simulink library "dynamicsLibrary"  (R2019a)
settings: Solver=ode45  StartTime=0.0  StopTime=10.0  RelTol=1e-3  EnableMultiTasking=on
undefined symbols (not defined in the file): Vehicle
settings Model: Creator=The MathWorks, Inc.  LastModifiedBy=yahyaaba
settings DataIOCC: LimitDataPoints=on  SaveFormat=Array  ReturnWorkspaceOutputs=off
settings OptimizationCC: LifeSpan=inf
settings DebuggingCC: UnderspecifiedInitializationDetection=Classic  MergeDetectMultiDrivingBlocksExec=none  SolverPrmCheckMsg=warning  AllowSymbolicDim=off  SFUnexpectedBacktrackingDiag=warning  SFNoUnconditionalDefaultTransitionDiag=warning  SFExecutionAtInitializationDiag=none  ArithmeticOperatorsInVariantConditions=warning
settings HardwareCC: ProdBitPerPointer=32  ProdBitPerSizeT=32  ProdBitPerPtrDiffT=32  ProdLargestAtomicFloat=None  ProdIntDivRoundTo=Undefined  ProdEndianess=Unspecified  ProdWordSize=32  ProdHWDeviceType=32-bit Generic
settings ModelReferenceCC: PropagateSignalLabelsOutOfModel=off
settings SFSimCC: SimUseLocalCustomCode=off
settings RTWCC: RTWUseLocalCustomCode=off
settings CodeAppCC: StateflowObjectComments=on
settings GRTTargetCC: TargetLangStandard=C89/C90 (ANSI)  GeneratePreprocessorConditionals=Disable all
settings ConfigComp: CovMetricSettings=dw  CovHtmlReporting=on  CovSaveCumulativeToWorkspaceVar=on  CovSaveSingleToWorkspaceVar=on  CovExternalEMLEnable=off  CovSFcnEnable=off

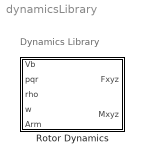
== system dynamicsLibrary ==
  note: Dynamics Library
  Rotor Dynamics : Subsystem  TreatAsAtomicUnit=on
      mask init:
      | aeroicon('aeroblk');
      settings: RTWFcnNameOpts=Use subsystem name  RTWFileNameOpts=Use function name

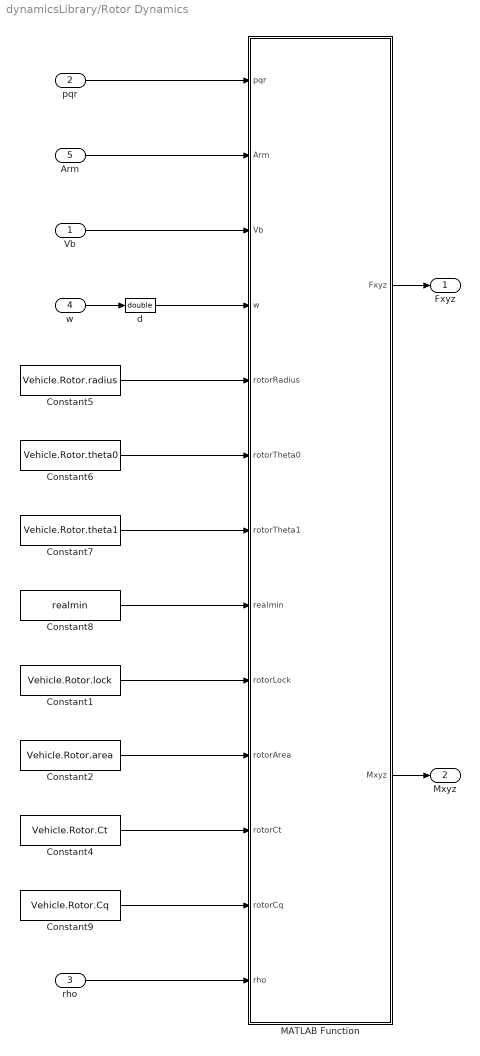
== system dynamicsLibrary/Rotor Dynamics ==
  Vb : Inport  PortDimensions=3
  pqr : Inport  Port=2  PortDimensions=3
  rho : Inport  Port=3  PortDimensions=1
  w : Inport  Port=4  PortDimensions=[1 1]
  Arm : Inport  Port=5  PortDimensions=[3 1]
  Constant1 : Constant  Value=Vehicle.Rotor.lock
  Constant2 : Constant  Value=Vehicle.Rotor.area
  Constant4 : Constant  Value=Vehicle.Rotor.Ct
  Constant5 : Constant  Value=Vehicle.Rotor.radius
  Constant6 : Constant  Value=Vehicle.Rotor.theta0
  Constant7 : Constant  Value=Vehicle.Rotor.theta1
  Constant8 : Constant  Value=realmin
  Constant9 : Constant  Value=Vehicle.Rotor.Cq
  MATLAB Function : MATLAB Function  TreatAsAtomicUnit=on
  d : DataTypeConversion  OutDataTypeStr=double
  Fxyz : Outport  PortDimensions=[3 1]
  Mxyz : Outport  Port=2  PortDimensions=[3 1]
  wires:
  Constant1/1 -> MATLAB Function/9(rotorLock)
  pqr/1 -> MATLAB Function/1(pqr)
  Arm/1 -> MATLAB Function/2(Arm)
  w/1 -> d/1
  MATLAB Function/1(Fxyz) -> Fxyz/1
  Constant7/1 -> MATLAB Function/7(rotorTheta1)
  rho/1 -> MATLAB Function/13(rho)
  Vb/1 -> MATLAB Function/3(Vb)
  Constant6/1 -> MATLAB Function/6(rotorTheta0)
  Constant4/1 -> MATLAB Function/11(rotorCt)
  d/1 -> MATLAB Function/4(w)
  Constant2/1 -> MATLAB Function/10(rotorArea)
  Constant9/1 -> MATLAB Function/12(rotorCq)
  Constant5/1 -> MATLAB Function/5(rotorRadius)
  Constant8/1 -> MATLAB Function/8(realmin)
  MATLAB Function/2(Mxyz) -> Mxyz/1

== matlab function dynamicsLibrary/Rotor Dynamics/MATLAB Function ==
  data: pqr input; Arm input; Vb input; w input; rotorRadius input; rotorTheta0 input; rotorTheta1 input; realmin input; rotorLock input; rotorArea input; rotorCt input; rotorCq input; rho input; Fxyz output; Mxyz output
function [Fxyz, Mxyz]  = rotorDynamics(pqr,Arm, Vb, w, rotorRadius, rotorTheta0, rotorTheta1, realmin, rotorLock, rotorArea, rotorCt, rotorCq, rho)

Vr = cross(pqr, Arm)+Vb;

Ic=Vr(3)/( abs(w)*rotorRadius );


mu= real( sqrt( sum(Vr(1:2).^2) ) )/ ( abs(w)*rotorRadius );

alphas=atan2(Ic,mu); % terminated



if mu~=0   
    tmp=[((8/3*rotorTheta0+2*rotorTheta1 )-Ic*2)/ (1./mu-0.5*mu); 0];
else
    tmp=[((8/3*rotorTheta0+2*rotorTheta1 )-Ic*2)/ (1./realmin-0.5*mu); 0];
end

j=atan2(Vr(2), Vr(1));

J=[[cos(j); sin(j)] [-sin(j); cos(j)] ];


beta=J.' * tmp;

tmp1=beta-( ((16/rotorLock)/abs(w)).*[pqr(2);pqr(1)] );


a1s=tmp1(1);
b1s=tmp1(2);


Fxyz=[sin(a1s)*-cos(b1s); sin(b1s); -cos(a1s)*cos(b1s)]* w.^2 * (rotorCt*rotorRadius^2*rotorArea) * rho ;

tau=cross(Arm, Fxyz);


out2=[0;0; rho*abs(w)*w*(-rotorCq*rotorRadius^3*rotorArea)];

Mxyz=tau+out2;
